simulink model "test"  (R2018a)
settings: Solver=VariableStepAuto  StartTime=0.0  StopTime=1  RelTol=1e-3
undefined symbols (not defined in the file): fdesignblkfcn, G1, G2, G3, G4, G5, G6, G7, G8, gcbh, get, T
libraries: dspsrcs4 x9, dspxfrm3 x2, dspobslib x2
(part 2 of 3)

== system test/Filter Bank /Filter 6/Bandpass Filter ==
  In : Inport
  Generated Filter Block : DiscreteFir  Tag=BlockMethodSubSystem  Coefficients=[0.000607647590175360518 0.000206090095044535421 6.32070585742618347e-05 -0.000169246908395596766 -0.000402577347030018916 -0.000536076896013370726 -0.000509633863550356444 -0.000341304998536757955 -0.000126290906658216995 1.03827066601906228e-05 -1.27259351147796766e-05 -0.000171126970283818394 -0.000323773063986194834 -0.000271106964411288638 0.000134059561458867935 0.00087427826617740513 0.00171536869741326331 0.0022605597953360302 0.0021071549211400596 0.00104973329233353342 -0.000765568289350088377 -0.00282053527372099454 -0.0043751846577421696 -0.00474619052960678113 -0.00360882802294115084 -0.0011834427684287714 0.00179317422444540131 0.00432368298057256815 0.00552951269840618216 0.00501842874823609994 0.00304789004409119916 0.000422885558803136428 -0.00184911949514523859 -0.00299469972593076686 -0.00280232079249016167 -0.00169018627341275597 -0.000473775947542854844 5.78103341194326594e-05 -0.000443552579410507364 -0.00168822728154093124 -0.00287543883520038858 -0.0030959702564114012 -0.0018191323598770908 0.000777255974324846848 0.00381272288372904843 0.00606375935352039888 0.0065223119839569587 0.00488673832961143782 0.00173960073646639611 -0.00169238928322594517 -0.00409496935999434548 -0.00467961527679951889 -0.00355047909047568775 -0.00163268882460580788 -0.000181508649258438635 -0.00011053611144375982 -0.00147229098395954472 -0.0033766914054368922 -0.00441286661207202467 -0.00339079579508019422 -3.91581706003813967e-05 0.00470887428145778941 0.00902341521609742979 0.0109744019444994248 0.00945297444500392547 0.00476745477243780812 -0.00140578818672822147 -0.0067323426465262055 -0.00927855227513746383 -0.00841328496115175545 -0.00509795406558999267 -0.00139162055451158757 0.000613526905867995288 -8.94268366715344164e-05 -0.00282474855760986169 -0.00550210798501878096 -0.00567380992376671865 -0.00189095275707261748 0.00532354030184395855 0.0134277422138286816 0.0188562838272313057 0.018655340922534229 0.0119942034085430832 0.000789633049189227107 -0.0109458599561518943 -0.0188145707387460462 -0.020044232378388753 -0.0148311709950778477 -0.00630352111533789231 0.000975708970731358621 0.00332540125655374262 -2.49245937322677716e-05 -0.00625677586351438327 -0.0101244152124268846 -0.00657410721325925058 0.0063304006983010818 0.0256131472667011605 0.0437777508307613944 0.0515157155527460331 0.0417751835533258439 0.0134838746648565169 -0.0268191231061600949 -0.0664377927042587163 -0.0907916785614623634 -0.0889862670960956115 -0.0584759427916168445 -0.00683011901805155239 0.0503152084541465539 0.0945239900709876069 0.111118716160494319 0.0945239900709876069 0.0503152084541465539 -0.00683011901805155239 -0.0584759427916168445 -0.0889862670960956115 -0.0907916785614623634 -0.0664377927042587163 -0.0268191231061600949 0.0134838746648565169 0.0417751835533258439 0.0515157155527460331 0.0437777508307613944 0.0256131472667011605 0.0063304006983010818 -0.00657410721325925058 -0.0101244152124268846 -0.00625677586351438327 -2.49245937322677716e-05 0.00332540125655374262 0.000975708970731358621 -0.00630352111533789231 -0.0148311709950778477 -0.020044232378388753 -0.0188145707387460462 -0.0109458599561518943 0.000789633049189227107 0.0119942034085430832 0.018655340922534229 0.0188562838272313057 0.0134277422138286816 0.00532354030184395855 -0.00189095275707261748 -0.00567380992376671865 -0.00550210798501878096 -0.00282474855760986169 -8.94268366715344164e-05 0.000613526905867995288 -0.00139162055451158757 -0.00509795406558999267 -0.00841328496115175545 -0.00927855227513746383 -0.0067323426465262055 -0.00140578818672822147 0.00476745477243780812 0.00945297444500392547 0.0109744019444994248 0.00902341521609742979 0.00470887428145778941 -3.91581706003813967e-05 -0.00339079579508019422 -0.00441286661207202467 -0.0033766914054368922 -0.00147229098395954472 -0.00011053611144375982 -0.000181508649258438635 -0.00163268882460580788 -0.00355047909047568775 -0.00467961527679951889 -0.00409496935999434548 -0.00169238928322594517 ...(+1167 chars)]  InputProcessing=Columns as channels (frame based)
  Out : Outport
  wires:
  In/1 -> Generated Filter Block/1
  Generated Filter Block/1 -> Out/1

== system test/Filter Bank /Filter 7/Bandpass Filter ==
  In : Inport
  Generated Filter Block : DiscreteFir  Tag=BlockMethodSubSystem  Coefficients=[0.000688747021894905889 2.18684298008015856e-05 -0.000747774121627521084 -0.000944058309513606591 -0.0003253492168160309 9.23101405120965485e-05 -0.000131668261710039206 0.000278299081757325871 0.00203685546617077794 0.00282127501297776626 -0.000224709806789325146 -0.00520584422999511177 -0.00594883627287124024 0.000104776300548475431 0.00699311488289822321 0.00678303313259411272 -0.000102973163323512827 -0.00534202521083943123 -0.00384222786058355031 0.000225635118397079837 0.000786570913460919751 -0.00113558835506687812 -0.000356549883511292831 0.00316551500606420452 0.00402210419483252021 0.000322671204025696797 -0.00302827437643997388 -0.00216241189084108009 -0.000100813788313752328 -0.000946319429482982534 -0.00249356303439283132 -0.000132893301647272187 0.00440682241811530574 0.00478680562478373157 0.000166602611108409172 -0.00313585876482802518 -0.00167151510761213767 1.82691025068816831e-05 -0.0021013983861952008 -0.00395901110293506858 -0.000207114547394701611 0.00567024530585669498 0.00573968097265152143 0.000174823472250806768 -0.00296323872407792347 -0.000848885771231672344 6.02451606138625724e-05 -0.00386543105769642436 -0.00596799938366046438 -0.000241959352823016387 0.00725476107922014279 0.00675905125520697651 0.000156525444502864661 -0.00239642366385430005 0.000584860770044941854 0.000116746090016668636 -0.00637431642816130468 -0.00864825281754785444 -0.000274770149259543229 0.00906406170058568321 0.00767549981510917429 0.000128325194659888349 -0.00109798340411188574 0.00298635822444113554 0.000172013986760184787 -0.00995471786868828978 -0.0122262860177205709 -0.000289429179599843146 0.0110718951047434951 0.00828444979299942583 8.00096111541152974e-05 0.00143940511550613237 0.0069799678032253917 0.000230656445653469946 -0.0152584825098764434 -0.0172511918860694773 -0.000290673659826494631 0.0133414677838347932 0.00830270700510185242 2.19011819696309385e-05 0.00630234256282785968 0.0139879881369137093 0.000280183979399447648 -0.0240273714837147996 -0.0252923712533665752 -0.000272683548033014929 0.0162592575259398707 0.00706560096826768826 -4.35748078964608848e-05 0.0169311165912110519 0.0289161122637894945 0.000315185308307668402 -0.0431671491461131721 -0.0431328019381585631 -0.000233050029664418762 0.0220958062178700232 0.00150542181965559411 -0.000114144512323115406 0.0556632812146515277 0.0889235674356774614 0.000335148073650662348 -0.151569396799215494 -0.17692677818321656 -0.000178950765438543047 0.204075838377702878 0.204075838377702878 -0.000178950765438543047 -0.17692677818321656 -0.151569396799215494 0.000335148073650662348 0.0889235674356774614 0.0556632812146515277 -0.000114144512323115406 0.00150542181965559411 0.0220958062178700232 -0.000233050029664418762 -0.0431328019381585631 -0.0431671491461131721 0.000315185308307668402 0.0289161122637894945 0.0169311165912110519 -4.35748078964608848e-05 0.00706560096826768826 0.0162592575259398707 -0.000272683548033014929 -0.0252923712533665752 -0.0240273714837147996 0.000280183979399447648 0.0139879881369137093 0.00630234256282785968 2.19011819696309385e-05 0.00830270700510185242 0.0133414677838347932 -0.000290673659826494631 -0.0172511918860694773 -0.0152584825098764434 0.000230656445653469946 0.0069799678032253917 0.00143940511550613237 8.00096111541152974e-05 0.00828444979299942583 0.0110718951047434951 -0.000289429179599843146 -0.0122262860177205709 -0.00995471786868828978 0.000172013986760184787 0.00298635822444113554 -0.00109798340411188574 0.000128325194659888349 0.00767549981510917429 0.00906406170058568321 -0.000274770149259543229 -0.00864825281754785444 -0.00637431642816130468 0.000116746090016668636 0.000584860770044941854 -0.00239642366385430005 0.000156525444502864661 0.00675905125520697651 0.00725476107922014279 -0.000241959352823016387 -0.00596799938366046438 -0.00386543105769642436 6.02451606138625724e-05 -0.000848885771231672344 -0.00296323872407792347 0.000174823472250806768 0.00573968097265152143 0.00567024530585669498 ...(+984 chars)]  InputProcessing=Columns as channels (frame based)
  Out : Outport
  wires:
  In/1 -> Generated Filter Block/1
  Generated Filter Block/1 -> Out/1

== system test/Filter Bank /Filter 8/Bandpass Filter ==
  In : Inport
  Generated Filter Block : DiscreteFir  Tag=BlockMethodSubSystem  Coefficients=[0.00208920521587915246 -0.00239512818882031209 -0.00053855600712965075 0.00150475259248641934 0.00252544250182454386 -0.00262685013507397373 -0.00682438869370431342 0.0130444383713146095 -0.00467990488077754934 -0.00666027455039981762 0.0065164932128488522 -0.001729553695465373 0.0027950984838265476 -0.00392121882782151248 0.000137629180377313461 0.000691755262694491112 0.00294733775033876894 -0.00196841445717181639 -0.00248992082802597988 0.0017519958426288815 0.00046966668933724748 0.00262630220439261791 -0.00459492818474551735 0.00106769995546806499 -0.000389444490693690399 0.0038542944042112481 -0.00236351548851125191 -0.00188112642215912135 0.000257224238094455951 0.00169589471518602508 0.00265878035526694121 -0.00473885524561892639 0.000805894918949866213 -0.00119578655816939298 0.00565818675776582573 -0.00335162697798689103 -0.00121382357210092972 -0.00163666245933176305 0.0034257953253684398 0.00255966812741642222 -0.00452860735243412835 -0.000172673285062963013 -0.00174515950402045128 0.00762753758969023869 -0.00427652780988023798 -0.000415142871464710037 -0.00434745674088348692 0.00594572238940444236 0.00198782770890439412 -0.00339539960772064281 -0.00235619635441489984 -0.00174154397900754031 0.00932818297228426609 -0.00456412086188246781 0.000211468997190310308 -0.00783040750598629036 0.00912027015947805379 0.00101066349951296286 -0.000993201992272878427 -0.00621406621928159274 -0.000933278796841543546 0.010374879780530635 -0.0035058074009965837 0.000183774544916749492 -0.0119932781167965165 0.0127164419702139927 -0.000118627653125519638 0.00306665921662160369 -0.0124560410028310802 0.00103531382505865003 0.0102247032262783432 0.000114107468776567908 -0.00138498443566570872 -0.0167418874624110751 0.0162963794100802369 -0.000676383865222395376 0.00932848769675900108 -0.0223771025899010684 0.0044915073428323047 0.00831785564204764148 0.00860697865906221923 -0.00610825532917689748 -0.0226525365322748432 0.0193817763974839519 0.00104923132526923502 0.0197960166547991728 -0.0404947799116348456 0.0104095040355148393 0.00325393347708273582 0.0303041591252078656 -0.019893795865867276 -0.0338370562033461705 0.021461701983966644 0.0127466721478665217 0.0484039343744557954 -0.100143205815215075 0.0276522419142769607 -0.0181644642821803294 0.171371970609715235 -0.150178366693390353 -0.218300812871885463 0.466638075069337244 -0.218300812871885463 -0.150178366693390353 0.171371970609715235 -0.0181644642821803294 0.0276522419142769607 -0.100143205815215075 0.0484039343744557954 0.0127466721478665217 0.021461701983966644 -0.0338370562033461705 -0.019893795865867276 0.0303041591252078656 0.00325393347708273582 0.0104095040355148393 -0.0404947799116348456 0.0197960166547991728 0.00104923132526923502 0.0193817763974839519 -0.0226525365322748432 -0.00610825532917689748 0.00860697865906221923 0.00831785564204764148 0.0044915073428323047 -0.0223771025899010684 0.00932848769675900108 -0.000676383865222395376 0.0162963794100802369 -0.0167418874624110751 -0.00138498443566570872 0.000114107468776567908 0.0102247032262783432 0.00103531382505865003 -0.0124560410028310802 0.00306665921662160369 -0.000118627653125519638 0.0127164419702139927 -0.0119932781167965165 0.000183774544916749492 -0.0035058074009965837 0.010374879780530635 -0.000933278796841543546 -0.00621406621928159274 -0.000993201992272878427 0.00101066349951296286 0.00912027015947805379 -0.00783040750598629036 0.000211468997190310308 -0.00456412086188246781 0.00932818297228426609 -0.00174154397900754031 -0.00235619635441489984 -0.00339539960772064281 0.00198782770890439412 0.00594572238940444236 -0.00434745674088348692 -0.000415142871464710037 -0.00427652780988023798 0.00762753758969023869 -0.00174515950402045128 -0.000172673285062963013 -0.00452860735243412835 0.00255966812741642222 0.0034257953253684398 -0.00163666245933176305 -0.00121382357210092972 -0.00335162697798689103 0.00565818675776582573 -0.00119578655816939298 0.000805894918949866213 -0.00473885524561892639 ...(+724 chars)]  InputProcessing=Columns as channels (frame based)
  Out : Outport
  wires:
  In/1 -> Generated Filter Block/1
  Generated Filter Block/1 -> Out/1
